simulink model "hexacopter_backup"  (R2023b)
settings: Solver=ode3  StartTime=0.0  StopTime=inf  FixedStep=0.005  RelTol=1e-3
values from neighbouring files (symbols this model uses):
  A = [zeros(4),eye(4) ... (first row only)    [hexacopter_params.m]
  B = [0 0 0 0 ... (first row only)    [hexa.m]    (also in hexacopter_params.m = [zeros(4))
  body_params = [L,b,d,m,Ix,Iy,Iz,J_T]    [hexacopter_params.m]
  C = eye(8)    [hexacopter_params.m]
  g = 9.82    [hexacopter_params.m]
  K = place(A', C', desired_poles)'    [hexacopter_params.m]
  m = 2.5    [hexacopter_params.m]
  Simulation_params = [g,K_phi,K_theta,K_psi,K_x,K_y,K_z]    [hexacopter_params.m]
  T = [1, 1, 1, 1, 1, 1 ... (first row only)    [hexacopter_params.m]
  T_inv = pinv(T)    [hexacopter_params.m]
libraries: slpidlib x8, simulink_extras x3, aerolibutil x2, vrlib x2
(part 2 of 2)

== matlab function hexacopter_backup/Subsystem/MATLAB Function ==
  data: x_hat input; params input; motorspeeds input; out output
function out = h(x_hat,params,motorspeeds)

Ix = params(5);
Iy = params(6);
Iz = params(7);
J_T = params(8);

g = 9.82;

phi_dot = x_hat(2);
theta_dot = x_hat(4);
psi_dot = x_hat(6);

Omega = motorspeeds(3)+motorspeeds(4)-motorspeeds(1)-motorspeeds(2);
max_omega = 1;  % Maximum yaw rate (in rad/s)
Omega = max(min(Omega, max_omega), -max_omega);  % Saturate Omega

out = [zeros(4,1);
       (theta_dot*psi_dot*(Iy-Iz)-J_T*theta_dot*Omega)/Ix;
       (phi_dot*psi_dot*(Iz-Ix)-J_T*phi_dot*Omega)/Iy;
       phi_dot*theta_dot*(Ix-Iy)/Iz;
       -g];

% out = zeros(8,1);

== matlab function hexacopter_backup/MATLAB Function1 ==
  data: u input; motorspeeds output; Thrust_matrix input
function motorspeeds = fcn(u, Thrust_matrix)


motorspeeds = quadprog(Thrust_matrix, u);
